simulink model "Simulation_I_controller"  (R2023a)
settings: Solver=VariableStepAuto  StartTime=0.0  StopTime=100  MaxStep=1e-3
settings Model: Creator=mazen  LastModifiedBy=mazen

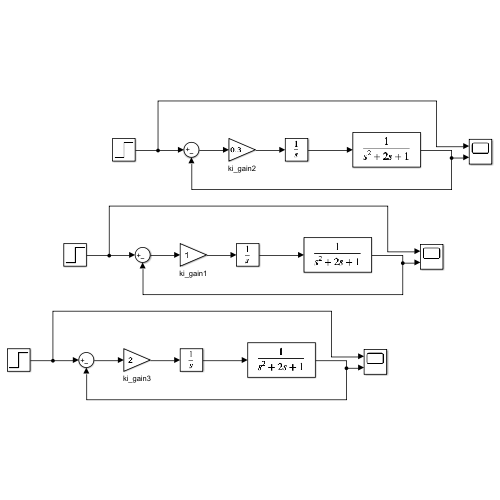
[thumbnail: Simulink's stored preview of the top-level diagram]
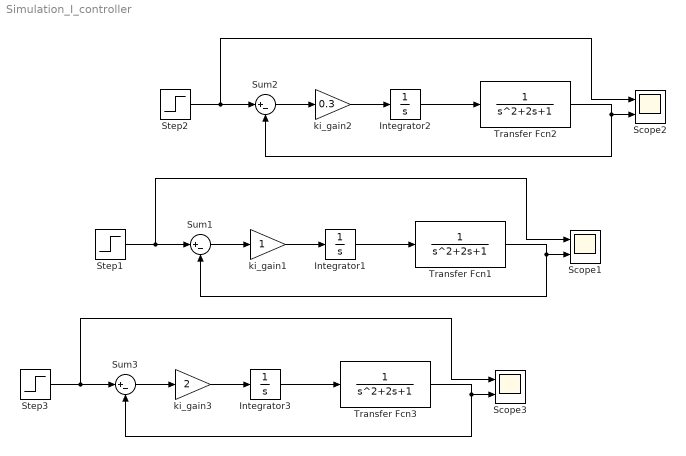
== system Simulation_I_controller ==
  Integrator1 : Integrator
  Integrator2 : Integrator
  Integrator3 : Integrator
  Scope1 : Scope  NumInputPorts=2
  Scope2 : Scope  NumInputPorts=2
  Scope3 : Scope  NumInputPorts=2
  Step1 : Step  SampleTime=0
  Step2 : Step  SampleTime=0
  Step3 : Step  SampleTime=0
  Sum1 : Sum  Inputs=|+-
  Sum2 : Sum  Inputs=|+-
  Sum3 : Sum  Inputs=|+-
  Transfer Fcn1 : TransferFcn
  Transfer Fcn2 : TransferFcn
  Transfer Fcn3 : TransferFcn
  ki_gain1 : Gain
  ki_gain2 : Gain  Gain=0.3
  ki_gain3 : Gain  Gain=2
  wires:
  Sum2/1 -> ki_gain2/1
  ki_gain2/1 -> Integrator2/1
  Integrator2/1 -> Transfer Fcn2/1
  Transfer Fcn2/1 -> Sum2/2, Scope2/2
  Step2/1 -> Scope2/1, Sum2/1
  Step1/1 -> Sum1/1, Scope1/1
  Transfer Fcn1/1 -> Scope1/2, Sum1/2
  Integrator1/1 -> Transfer Fcn1/1
  ki_gain1/1 -> Integrator1/1
  Sum1/1 -> ki_gain1/1
  Sum3/1 -> ki_gain3/1
  ki_gain3/1 -> Integrator3/1
  Integrator3/1 -> Transfer Fcn3/1
  Transfer Fcn3/1 -> Sum3/2, Scope3/2
  Step3/1 -> Scope3/1, Sum3/1
